simulink library "aplib"  (Simulink 10.0)
settings: Solver=VariableStepAuto  StartTime=0.0  StopTime=10.0  RelTol=1e-3
undefined symbols (not defined in the file): Aail, Aelv, Arud, Bail, Belv, Brud, Cail, CD, Celv, Crud, Dail, Delv, Drud, gamgs, HRW, Sgs, Sloc, uaero0, uprop0, xdot0, xgs, xinco, xloc, ymod1A, ymod1S, ymod2A, ymod2S, yrefA, yrefS
libraries: fdctools x42, navlib1 x8, navlib2 x2, wndlib1 x1, wndlib2 x1
(part 2 of 2)

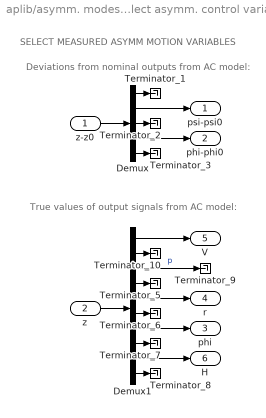
== system aplib/asymm. modes/Select asymm. control variables ==
  note: SELECT MEASURED ASYMM MOTION VARIABLES
  note: Deviations from nominal outputs from AC model:
  note: True values of output signals from AC model:
  z-z0 : Inport
  z : Inport  Port=2
  Demux : Demux  Outputs=[6 1 1 1 4]
  Demux1 : Demux  Outputs=[1 2 1 1 1 2 1 2 1 1]
  Terminator_{1..3,5..10} (9 alike) : Terminator
  psi-psi0 : Outport
  phi-phi0 : Outport  Port=2
  phi : Outport  Port=3
  r : Outport  Port=4
  V : Outport  Port=5
  H : Outport  Port=6
  wires:
  Demux/5 -> Terminator_3/1
  z-z0/1 -> Demux/1
  Demux/2 -> psi-psi0/1
  Demux/4 -> phi-phi0/1
  Demux/1 -> Terminator_1/1
  Demux/3 -> Terminator_2/1
  Demux1/9 -> H/1
  z/1 -> Demux1/1
  Demux1/3 -> Terminator_9/1  "p"
  Demux1/5 -> r/1
  Demux1/7 -> phi/1
  Demux1/2 -> Terminator_10/1
  Demux1/4 -> Terminator_5/1
  Demux1/6 -> Terminator_6/1
  Demux1/8 -> Terminator_7/1
  Demux1/10 -> Terminator_8/1
  Demux1/1 -> V/1

== system aplib/asymm. modes/Select asymm. mode-controller signals ==
  note: SELECT ASYMM MODE
      | (on/off flags denoted by '?')
  note: SELECT ASYMM REFERENCE SIGNALS
  ymode : Inport
  yref : Inport  Port=2
  Demux : Demux  Outputs=[5 1 1 1 1 1]
  Demux1 : Demux  Outputs=[3 1 1]
  Terminator_1 : Terminator
  Terminator_2 : Terminator
  Asymm. mode? : Outport
  Asymm. outer loop? : Outport  Port=2
  Dphir (RAH) : Outport  Port=3
  HH? : Outport  Port=4
  Dpsir (HH) : Outport  Port=5
  NAV? : Outport  Port=6
  LOC coupled? : Outport  Port=7
  wires:
  ymode/1 -> Demux/1
  Demux/2 -> Asymm. mode?/1
  Demux/3 -> Asymm. outer loop?/1
  Demux/4 -> HH?/1
  Demux/5 -> NAV?/1
  Demux/6 -> LOC coupled?/1
  Demux/1 -> Terminator_1/1
  yref/1 -> Demux1/1
  Demux1/2 -> Dphir (RAH)/1
  Demux1/3 -> Dpsir (HH)/1
  Demux1/1 -> Terminator_2/1

== system aplib/asymm. modes/t ==

== system aplib/delay & limiters/t ==

== system aplib/mode controller/t ==

== system aplib/symm. modes/ALH ==
  note: Altitude Hold mode
  ALH? : Inport
  DHr (ALH) : Inport  Port=2
  H-H0 : Inport  Port=3
  V : Inport  Port=4
  KH : fdctools/Scheduled Gain  K=(-1.0*10^(-4)*u[1]^2 + 0.015*u[1] - 0.5975)*(pi/180)
  On/Off : fdctools/On//off switch
  Sum : Sum  Inputs=+-  SaturateOnIntegerOverflow=on  InputSameDT=on  OutDataTypeStr=Inherit: Same as first input
  Dthetar (ALH) : Outport
  wires:
  V/1 -> KH/1
  Sum/1 -> KH/2
  KH/1 -> On/Off/2
  ALH?/1 -> On/Off/1
  DHr (ALH)/1 -> Sum/1
  On/Off/1 -> Dthetar (ALH)/1
  H-H0/1 -> Sum/2

== system aplib/symm. modes/ALS ==
  note: Altitude Select Mode
  ALS? : Inport
  DHdot r (ALS) : Inport  Port=2
  Hdot-Hdot0 : Inport  Port=3
  V : Inport  Port=4
  KHdot : fdctools/Scheduled Gain  K=(-3.875*10^(-4)*u[1]^2 + 0.04025*u[1] - 1.1041)*(pi/180)
  On/Off : fdctools/On//off switch
  Sum : Sum  Inputs=+-  SaturateOnIntegerOverflow=on  InputSameDT=on  OutDataTypeStr=Inherit: Same as first input
  filter : TransferFcn  Denominator=[1 0.15]
  Dthetar (ALS) : Outport
  wires:
  V/1 -> KHdot/1
  Hdot-Hdot0/1 -> Sum/2
  KHdot/1 -> On/Off/2
  ALS?/1 -> On/Off/1
  DHdot r (ALS)/1 -> Sum/1
  On/Off/1 -> Dthetar (ALS)/1
  Sum/1 -> filter/1
  filter/1 -> KHdot/2

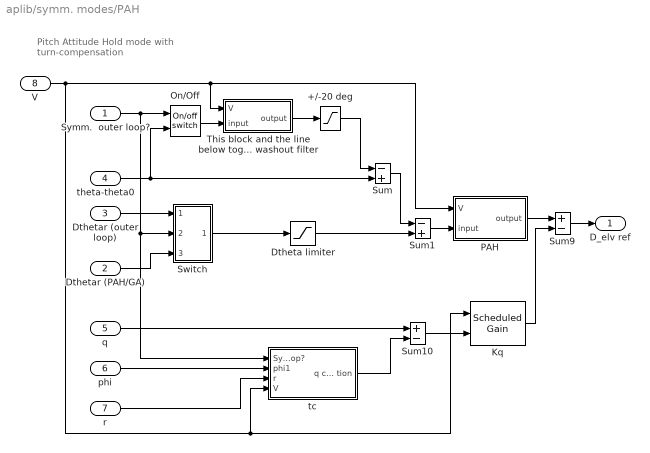
== system aplib/symm. modes/PAH ==
  note: Pitch Attitude Hold mode
      | with turn-compensation
  Symm.  outer loop? : Inport
  Dthetar (PAH/GA) : Inport  Port=2
  Dthetar (outer loop) : Inport  Port=3
  theta-theta0 : Inport  Port=4
  q : Inport  Port=5
  phi : Inport  Port=6
  r : Inport  Port=7
  V : Inport  Port=8
  +/-20 deg : Saturate  UpperLimit=20*(pi/180)  LowerLimit=-20*(pi/180)
  Dtheta limiter : Saturate  UpperLimit=18*(pi/180)  LowerLimit=-8*(pi/180)
  Kq : fdctools/Scheduled Gain  K=-4.75*10^(-4)*u[1]^2 +0.0540*u[1] - 1.5931
  On/Off : fdctools/On//off switch
  PAH : Subsystem
      mask Display: disp('PAH (limited \n PI controller)')
  Sum : Sum  Inputs=-+  SaturateOnIntegerOverflow=on  InputSameDT=on  OutDataTypeStr=Inherit: Same as first input
  Sum1 : Sum  Inputs=-+  SaturateOnIntegerOverflow=on  InputSameDT=on  OutDataTypeStr=Inherit: Same as first input
  Sum10 : Sum  Inputs=+-  SaturateOnIntegerOverflow=on  InputSameDT=on  OutDataTypeStr=Inherit: Same as first input
  Sum9 : Sum  Inputs=+-  SaturateOnIntegerOverflow=on  InputSameDT=on  OutDataTypeStr=Inherit: Same as first input
  Switch : Subsystem
      mask Display: plot(0,0,100,100,[100,70,40,0],[50,50,80,80],[40,0],[20,20],[29,29,0],[64,50,50],[29,29],[36,50],[40,40,41,40,39,40],[80,82,80,78,80,82],[40,40,41,40,39,40],[19,21,20,18,20,23])
  This block and the line below together form a washout filter : Subsystem
      mask Display: disp('Kd/(s+Kd)')
  tc : Subsystem
      mask Display: disp('Turn\nCompensator')
  D_elv ref : Outport
  wires:
  Dthetar (outer loop)/1 -> Switch/1(Dthetar (outer loop))
  Switch/1(Dthetar) -> Dtheta limiter/1
  Sum1/1 -> PAH/2(input)
  Dtheta limiter/1 -> Sum1/2
  PAH/1(output) -> Sum9/1
  Kq/1 -> Sum9/2
  Sum/1 -> Sum1/1
  +/-20 deg/1 -> Sum/1
  theta-theta0/1 -> Sum/2, On/Off/2
  Dthetar (PAH/GA)/1 -> Switch/3(Dthetar (PAH/GA))
  r/1 -> tc/3(r)
  phi/1 -> tc/2(phi1)
  Sum10/1 -> Kq/2
  q/1 -> Sum10/1
  tc/1(q correc- tion) -> Sum10/2
  Sum9/1 -> D_elv ref/1
  Symm.  outer loop?/1 -> On/Off/1, tc/1(Symm. outer loop?), Switch/2(Symm.  outer loop?)
  This block and the line below together form a washout filter/1(output) -> +/-20 deg/1
  On/Off/1 -> This block and the line below together form a washout filter/2(input)
  V/1 -> Kq/1, tc/4(V), PAH/1(V), This block and the line below together form a washout filter/1(V)

== system aplib/symm. modes/Select symm control variables ==
  note: SELECT SYMMETRICAL CONTROL VARIABLES.
  note: True values of output signals from AC model:
  note: Deviations from nominal outputs from AC model:
  z-z0 : Inport
  z : Inport  Port=2
  Demux : Demux  Outputs=[7 1 3 1 1]
  Demux1 : Demux  Outputs=[1 3 1 1 2 1 2 1 1]
  Terminator_{1..6} (6 alike) : Terminator
  Hdot-Hdot0 : Outport
  H-H0 : Outport  Port=2
  theta-theta0 : Outport  Port=3
  q : Outport  Port=4
  phi : Outport  Port=5
  r : Outport  Port=6
  V : Outport  Port=7
  H : Outport  Port=8
  wires:
  Demux/1 -> Terminator_1/1
  z-z0/1 -> Demux/1
  Demux/3 -> Terminator_2/1
  Demux/5 -> Hdot-Hdot0/1
  Demux/4 -> H-H0/1
  Demux/2 -> theta-theta0/1
  Demux1/1 -> V/1
  z/1 -> Demux1/1
  Demux1/2 -> Terminator_3/1
  Demux1/5 -> Terminator_4/1
  Demux1/7 -> Terminator_5/1
  Demux1/9 -> Terminator_6/1
  Demux1/4 -> r/1
  Demux1/6 -> phi/1
  Demux1/8 -> H/1
  Demux1/3 -> q/1

== system aplib/symm. modes/Select symm. mode- controller signals ==
  note: SELECT SYMMETRICAL MODE
      | (on/off flags denoted by '?')
  note: SELECT SYMM REFERENCE SIGNALS
  ymode : Inport
  yref : Inport  Port=2
  Demux : Demux  Outputs=[1 1 1 1 1 5]
  Demux1 : Demux  Outputs=[1 1 1 2]
  Terminator_1 : Terminator
  Terminator_2 : Terminator
  Symm. mode? : Outport
  Symm. outer loop? : Outport  Port=2
  Dthetar (PAH) : Outport  Port=3
  ALS? : Outport  Port=4
  DHdot r (ALS) : Outport  Port=5
  ALH? : Outport  Port=6
  DHr (ALH) : Outport  Port=7
  GS coupled? : Outport  Port=8
  wires:
  Demux1/4 -> Terminator_2/1
  Demux1/3 -> DHdot r (ALS)/1
  Demux1/2 -> DHr (ALH)/1
  Demux1/1 -> Dthetar (PAH)/1
  yref/1 -> Demux1/1
  Demux/5 -> GS coupled?/1
  Demux/4 -> ALS?/1
  Demux/3 -> ALH?/1
  Demux/1 -> Symm. mode?/1
  Demux/2 -> Symm. outer loop?/1
  ymode/1 -> Demux/1
  Demux/6 -> Terminator_1/1

== system aplib/symm. modes/t ==

== system aplib/Asymm. modes/RAH/RAH ==
  note: PI controller for RAH
  V : Inport
  input u : Inport  Port=2
  +/-1V : Integrator  LimitOutput=on  UpperSaturationLimit=1*pi/180  LowerSaturationLimit=-1*pi/180
  +/-3.75V : Saturate  UpperLimit=3.75*pi/180  LowerLimit=-3.75*pi/180
  Ki : Gain  Gain=0.25  SaturateOnIntegerOverflow=on  OutDataTypeStr=Inherit: Same as input  ParamDataTypeStr=Inherit: Same as input
  Kphi : fdctools/Scheduled Gain  K=9.75*10^(-4)*u[1]^2-0.108*u[1]+2.335625
  Sum : Sum  SaturateOnIntegerOverflow=on  InputSameDT=on  OutDataTypeStr=Inherit: Same as first input
  output y : Outport
  wires:
  input u/1 -> Kphi/2
  Kphi/1 -> +/-3.75V/1
  V/1 -> Kphi/1
  +/-3.75V/1 -> Ki/1, Sum/1
  +/-1V/1 -> Sum/2
  Ki/1 -> +/-1V/1
  Sum/1 -> output y/1

== system aplib/Asymm. modes/RAH/Switch ==
  Dphir (outer loop) : Inport
  Asymm.  outer loop? : Inport  Port=2
  Dphir (RAH) : Inport  Port=3
  Sum2 : Sum  Inputs=-+  SaturateOnIntegerOverflow=on  InputSameDT=on  OutDataTypeStr=Inherit: Same as first input
  Switch : Switch  SaturateOnIntegerOverflow=on  InputSameDT=on
  const : Constant  Value=0.5
  Dphir : Outport
  wires:
  Dphir (outer loop)/1 -> Switch/1
  Dphir (RAH)/1 -> Switch/3
  Sum2/1 -> Switch/2
  const/1 -> Sum2/1
  Switch/1 -> Dphir/1
  Asymm.  outer loop?/1 -> Sum2/2

== system aplib/Sensors; subtract initial conditions/H/4ft quantizer ==
  In1 : Inport
  4ft quantizer : Fcn  Expr=u-rem(u,q)
  Out1 : Outport
  wires:
  In1/1 -> 4ft quantizer/1
  4ft quantizer/1 -> Out1/1

== system aplib/Symm. modes/PAH/PAH ==
  note: PI controller for PAH
  V : Inport
  input : Inport  Port=2
  +/- 10 V : Integrator  LimitOutput=on  UpperSaturationLimit=10*pi/180  LowerSaturationLimit=-10*pi/180
  +/- 2 V : Saturate  UpperLimit=2*pi/180  LowerLimit=-2*pi/180
  Ki : Gain  Gain=0.5  SaturateOnIntegerOverflow=on  OutDataTypeStr=Inherit: Same as input  ParamDataTypeStr=Inherit: Same as input
  Ktheta : fdctools/Scheduled Gain  K=-1.375*10^(-3)*u[1]^2 + 0.1575*u[1] - 4.8031
  Sum : Sum  SaturateOnIntegerOverflow=on  InputSameDT=on  OutDataTypeStr=Inherit: Same as first input
  output : Outport
  wires:
  Ki/1 -> +/- 10 V/1
  +/- 2 V/1 -> Ki/1, Sum/1
  +/- 10 V/1 -> Sum/2
  input/1 -> Ktheta/2
  V/1 -> Ktheta/1
  Sum/1 -> output/1
  Ktheta/1 -> +/- 2 V/1

== system aplib/Symm. modes/PAH/Switch ==
  Dthetar (outer loop) : Inport
  Symm.  outer loop? : Inport  Port=2
  Dthetar (PAH/GA) : Inport  Port=3
  Sum2 : Sum  Inputs=-+  SaturateOnIntegerOverflow=on  InputSameDT=on  OutDataTypeStr=Inherit: Same as first input
  Switch : Switch  SaturateOnIntegerOverflow=on  InputSameDT=on
  const : Constant  Value=0.5
  Dthetar : Outport
  wires:
  Switch/1 -> Dthetar/1
  Sum2/1 -> Switch/2
  Dthetar (PAH/GA)/1 -> Switch/3
  Dthetar (outer loop)/1 -> Switch/1
  const/1 -> Sum2/1
  Symm.  outer loop?/1 -> Sum2/2

== system aplib/Symm. modes/PAH/This block and the line below together form a washout filter ==
  note: Washout filter for PAH
  V : Inport
  input : Inport  Port=2
  1/s : Integrator
  Kd : fdctools/Scheduled Gain  K=-2.5*10^(-3)*u[1]+0.2875
  Sum : Sum  Inputs=+-  SaturateOnIntegerOverflow=on  InputSameDT=on  OutDataTypeStr=Inherit: Same as first input
  output : Outport
  wires:
  1/s/1 -> Kd/2
  Sum/1 -> 1/s/1
  Kd/1 -> output/1, Sum/2
  V/1 -> Kd/1
  input/1 -> Sum/1

== system aplib/Symm. modes/PAH/tc ==
  note: Turn-compensator
  Symm. outer loop? : Inport
  phi1 : Inport  Port=2
  r : Inport  Port=3
  V : Inport  Port=4
  Mux : Mux  Inputs=3
  "Turncomp. ALH (ALS, GS)" : Fcn  Expr=u[2]*tan(u[3]) + (0.03*u[1]+0.25)*((1/cos(u[3]+0.03491))-1)
  Turncomp. PAH : Fcn  Expr=u[2]*tan(u[3]) + (5.0*10^(-4)*u[1]^2 - 0.03*u[1] + 0.9375)*((1/cos(u[3])) - 1)
  switch : Switch  SaturateOnIntegerOverflow=on  InputSameDT=on
  q correc- tion : Outport
  wires:
  switch/1 -> q correc- tion/1
  Symm. outer loop?/1 -> switch/2
  phi1/1 -> Mux/3
  r/1 -> Mux/2
  "Turncomp. ALH (ALS, GS)"/1 -> switch/3
  V/1 -> Mux/1
  Mux/1 -> "Turncomp. ALH (ALS, GS)"/1, Turncomp. PAH/1
  Turncomp. PAH/1 -> switch/1

== system aplib/asymm. modes/RAH/RAH ==
  note: PI controller for RAH
  V : Inport
  input u : Inport  Port=2
  +/-1V : Integrator  LimitOutput=on  UpperSaturationLimit=1*pi/180  LowerSaturationLimit=-1*pi/180
  +/-3.75V : Saturate  UpperLimit=3.75*pi/180  LowerLimit=-3.75*pi/180
  Ki : Gain  Gain=0.25  SaturateOnIntegerOverflow=on  OutDataTypeStr=Inherit: Same as input  ParamDataTypeStr=Inherit: Same as input
  Kphi : fdctools/Scheduled Gain  K=9.75*10^(-4)*u[1]^2-0.108*u[1]+2.335625
  Sum : Sum  SaturateOnIntegerOverflow=on  InputSameDT=on  OutDataTypeStr=Inherit: Same as first input
  output y : Outport
  wires:
  input u/1 -> Kphi/2
  Kphi/1 -> +/-3.75V/1
  V/1 -> Kphi/1
  +/-3.75V/1 -> Ki/1, Sum/1
  +/-1V/1 -> Sum/2
  Ki/1 -> +/-1V/1
  Sum/1 -> output y/1

== system aplib/asymm. modes/RAH/Switch ==
  Dphir (outer loop) : Inport
  Asymm.  outer loop? : Inport  Port=2
  Dphir (RAH) : Inport  Port=3
  Sum2 : Sum  Inputs=-+  SaturateOnIntegerOverflow=on  InputSameDT=on  OutDataTypeStr=Inherit: Same as first input
  Switch : Switch  SaturateOnIntegerOverflow=on  InputSameDT=on
  const : Constant  Value=0.5
  Dphir : Outport
  wires:
  Dphir (outer loop)/1 -> Switch/1
  Dphir (RAH)/1 -> Switch/3
  Sum2/1 -> Switch/2
  const/1 -> Sum2/1
  Switch/1 -> Dphir/1
  Asymm.  outer loop?/1 -> Sum2/2

== system aplib/symm. modes/PAH/PAH ==
  note: PI controller for PAH
  V : Inport
  input : Inport  Port=2
  +/- 10 V : Integrator  LimitOutput=on  UpperSaturationLimit=10*pi/180  LowerSaturationLimit=-10*pi/180
  +/- 2 V : Saturate  UpperLimit=2*pi/180  LowerLimit=-2*pi/180
  Ki : Gain  Gain=0.5  SaturateOnIntegerOverflow=on  OutDataTypeStr=Inherit: Same as input  ParamDataTypeStr=Inherit: Same as input
  Ktheta : fdctools/Scheduled Gain  K=-1.375*10^(-3)*u[1]^2 + 0.1575*u[1] - 4.8031
  Sum : Sum  SaturateOnIntegerOverflow=on  InputSameDT=on  OutDataTypeStr=Inherit: Same as first input
  output : Outport
  wires:
  Ki/1 -> +/- 10 V/1
  +/- 2 V/1 -> Ki/1, Sum/1
  +/- 10 V/1 -> Sum/2
  input/1 -> Ktheta/2
  V/1 -> Ktheta/1
  Sum/1 -> output/1
  Ktheta/1 -> +/- 2 V/1

== system aplib/symm. modes/PAH/Switch ==
  Dthetar (outer loop) : Inport
  Symm.  outer loop? : Inport  Port=2
  Dthetar (PAH/GA) : Inport  Port=3
  Sum2 : Sum  Inputs=-+  SaturateOnIntegerOverflow=on  InputSameDT=on  OutDataTypeStr=Inherit: Same as first input
  Switch : Switch  SaturateOnIntegerOverflow=on  InputSameDT=on
  const : Constant  Value=0.5
  Dthetar : Outport
  wires:
  Switch/1 -> Dthetar/1
  Sum2/1 -> Switch/2
  Dthetar (PAH/GA)/1 -> Switch/3
  Dthetar (outer loop)/1 -> Switch/1
  const/1 -> Sum2/1
  Symm.  outer loop?/1 -> Sum2/2

== system aplib/symm. modes/PAH/This block and the line below together form a washout filter ==
  note: Washout filter for PAH
  V : Inport
  input : Inport  Port=2
  1/s : Integrator
  Kd : fdctools/Scheduled Gain  K=-2.5*10^(-3)*u[1]+0.2875
  Sum : Sum  Inputs=+-  SaturateOnIntegerOverflow=on  InputSameDT=on  OutDataTypeStr=Inherit: Same as first input
  output : Outport
  wires:
  1/s/1 -> Kd/2
  Sum/1 -> 1/s/1
  Kd/1 -> output/1, Sum/2
  V/1 -> Kd/1
  input/1 -> Sum/1

== system aplib/symm. modes/PAH/tc ==
  note: Turn-compensator
  Symm. outer loop? : Inport
  phi1 : Inport  Port=2
  r : Inport  Port=3
  V : Inport  Port=4
  Mux : Mux  Inputs=3
  "Turncomp. ALH (ALS, GS)" : Fcn  Expr=u[2]*tan(u[3]) + (0.03*u[1]+0.25)*((1/cos(u[3]+0.03491))-1)
  Turncomp. PAH : Fcn  Expr=u[2]*tan(u[3]) + (5.0*10^(-4)*u[1]^2 - 0.03*u[1] + 0.9375)*((1/cos(u[3])) - 1)
  switch : Switch  SaturateOnIntegerOverflow=on  InputSameDT=on
  q correc- tion : Outport
  wires:
  switch/1 -> q correc- tion/1
  Symm. outer loop?/1 -> switch/2
  phi1/1 -> Mux/3
  r/1 -> Mux/2
  "Turncomp. ALH (ALS, GS)"/1 -> switch/3
  V/1 -> Mux/1
  Mux/1 -> "Turncomp. ALH (ALS, GS)"/1, Turncomp. PAH/1
  Turncomp. PAH/1 -> switch/1
